simulink library "Enrg_conv_El_to_Mec_Bosch"  (R2016a)
settings: Solver=ode1  StartTime=0.0  StopTime=Inf  FixedStep=0.001  RelTol=1e-3
undefined symbols (not defined in the file): drvEmot_RefTqeMOT, FirstDrivenAxle_FirstDrivenAxleNoOfEmot, FMIKit, SecondDrivenAxle_SecondDrivenAxleNoOfEmot
libraries: Enrg_conv_El_to_Mec_Bosch x13, Electrical_converter x8
(part 2 of 5)

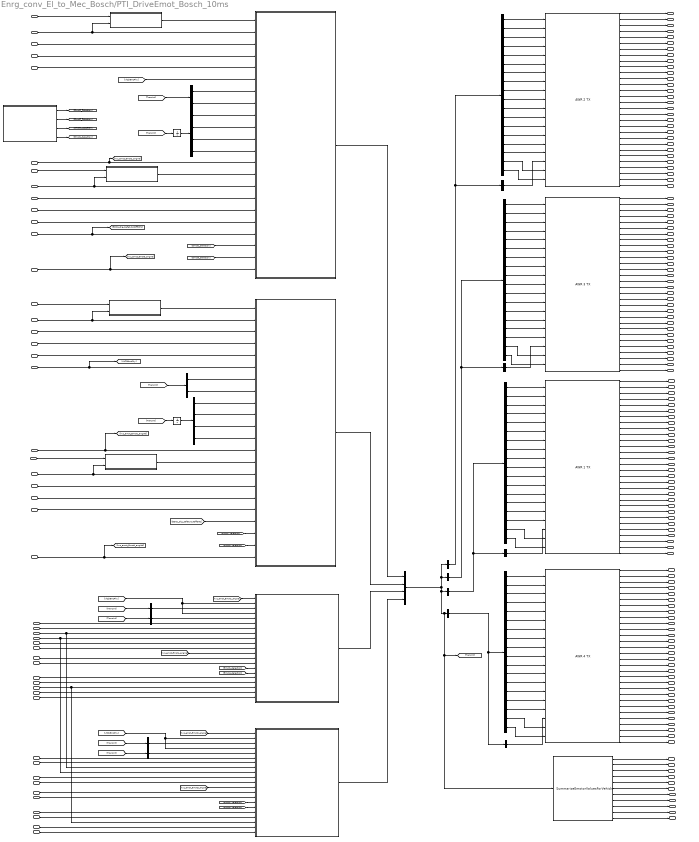
== system Enrg_conv_El_to_Mec_Bosch/PTI_DriveEmot_Bosch_10ms ==
  vltZkBmsPhy : Inport
  HVFreigabeHW1_SiRelay_D : Inport  Port=2
  HVFreigabeHW4_SiRelay_D : Inport  Port=3
  edcu_EMD1_CMD_ClearErrors : Inport  Port=4
  edcu_EMD1_CMD_ControlMode : Inport  Port=5
  edcu_EMD1_CMD_SpeedRefLim : Inport  Port=6
  pti_tqDesired_PTI1 : Inport  Description=[Nm]  Port=7
      settings: AttributesFormatString=%<Description>
  edcu_EMD4_CMD_ClearErrors : Inport  Port=8
  edcu_EMD4_CMD_ControlMode : Inport  Port=9
  edcu_EMD4_CMD_SpeedRefLim : Inport  Port=10
  pti_tqDesired_PTI4 : Inport  Description=[Nm]  Port=11
      settings: AttributesFormatString=%<Description>
  HVFreigabeHW2_SiRelay_D : Inport  Port=12
  HVFreigabeHW3_SiRelay_D : Inport  Port=13
  edcu_EMD2_CMD_ClearErrors : Inport  Port=14
  edcu_EMD2_CMD_ControlMode : Inport  Port=15
  edcu_EMD2_CMD_SpeedRefLim : Inport  Port=16
  pti_tqDesired_PTI2 : Inport  Description=[Nm]  Port=17
      settings: AttributesFormatString=%<Description>
  edcu_EMD3_CMD_ClearErrors : Inport  Port=18
  edcu_EMD3_CMD_ControlMode : Inport  Port=19
  edcu_EMD3_CMD_SpeedRefLim : Inport  Port=20
  pti_tqDesired_PTI3 : Inport  Description=[Nm]  Port=21
      settings: AttributesFormatString=%<Description>
  EDCU_Dig_SafetyCutOffDG1 : Inport  Port=22
  hvs_driveInverter1_switching_frequency : Inport  Port=23
  hvs_driveInverter2_switching_frequency : Inport  Port=24
  hvs_driveInverter3_switching_frequency : Inport  Port=25
  hvs_driveInverter4_switching_frequency : Inport  Port=26
  hvs_emot_Emot1_angVel : Inport  Port=27
  hvs_emot_Emot2_angVel : Inport  Port=28
  hvs_emot_Emot3_angVel : Inport  Port=29
  hvs_emot_Emot4_angVel : Inport  Port=30
  hvs_driveInverter_coolant_temperature : Inport  Port=31
  hvs_drvEmot1_Oil_Temperature : Inport  Port=32
  hvs_drvEmot1_Coolant_Temperature : Inport  Port=33
  hvs_drvEmot4Oil_Temperature : Inport  Port=34
  hvs_drvEmot4_Coolant_Temperature : Inport  Port=35
  hvs_drvEmot2_Oil_Temperature : Inport  Port=36
  hvs_drvEmot2_Coolant_Temperature : Inport  Port=37
  hvs_drvEmot3Oil_Temperature : Inport  Port=38
  hvs_drvEmot3_Coolant_Temperature : Inport  Port=39
  hvs_drvEmot_Ambient_Temperature : Inport  Port=40
  hvs_drvEmot1CoolantFlow_vdot : Inport  Port=41
  hvs_drvEmot1OilFlow_vdot : Inport  Port=42
  hvs_driveInverterCoolantFlow_vdot : Inport  Port=43
  hvs_drvEmot4CoolantFlow_vdot : Inport  Port=44
  hvs_drvEmot4OilFlow_vdot : Inport  Port=45
  hvs_drvEmot2CoolantFlow_vdot : Inport  Port=46
  hvs_drvEmot2OilFlow_vdot : Inport  Port=47
  hvs_drvEmot3CoolantFlow_vdot : Inport  Port=48
  hvs_drvEmot3OilFlow_vdot : Inport  Port=49
  AWR 1 TX1 : Enrg_conv_El_to_Mec_Bosch/PTI_DriveEmot_Bosch/AWR 1 TX
  AWR 2 TX1 : Enrg_conv_El_to_Mec_Bosch/PTI_DriveEmot_Bosch/AWR 2 TX
  AWR 3 TX1 : Enrg_conv_El_to_Mec_Bosch/PTI_DriveEmot_Bosch/AWR 3 TX
  AWR 4 TX1 : Enrg_conv_El_to_Mec_Bosch/PTI_DriveEmot_Bosch/AWR 4 TX
  AWR1_4 : Subsystem
  AWR2_3 : Subsystem
  Bus Selector21 : BusSelector  OutputSignals=EMD2_ACT_DcLinkVoltage,EMD_ACT_DigitalInput1,EMD_ACT_MaximumAvailableTorque,EMD_ACT_DcLinkPower,EMD_ACT_MotorSpeed,EMD_ACT_MotorTorque,EMD_ACT_InverterState,EMD_ACT_ReferenceTorqueLimited,drvEmot_T_Stator,drvEmot_T_Rotor,Inv_Ploss,mot_Ploss,uStator,iStator,modIdx,cosPhi,wasteHeat_coolant,wasteHeat_oil
  Bus Selector22 : BusSelector  OutputSignals=EMD1_ACT_DcLinkVoltage,EMD_ACT_DigitalInput1,EMD_ACT_MaximumAvailableTorque,EMD_ACT_DcLinkPower,EMD_ACT_MotorSpeed,EMD_ACT_MotorTorque,EMD_ACT_InverterState,EMD_ACT_ReferenceTorqueLimited,drvEmot_T_Stator,drvEmot_T_Rotor,Inv_Ploss,mot_Ploss,uStator,iStator,modIdx,cosPhi,wasteHeat_coolant,wasteHeat_oil
  Bus Selector23 : BusSelector  OutputSignals=EMD4_ACT_DcLinkVoltage,EMD_ACT_DigitalInput1,EMD_ACT_MaximumAvailableTorque,EMD_ACT_DcLinkPower,EMD_ACT_MotorSpeed,EMD_ACT_MotorTorque,EMD_ACT_InverterState,EMD_ACT_ReferenceTorqueLimited,drvEmot_T_Stator,drvEmot_T_Rotor,Inv_Ploss,mot_Ploss,uStator,iStator,modIdx,cosPhi,wasteHeat_coolant,wasteHeat_oil
  Bus Selector{24..27} (4 alike) : BusSelector  OutputSignals=driveInverter_Temperatures  OutputAsBus=on
  Bus Selector28 : BusSelector  OutputSignals=EMD3_ACT_DcLinkVoltage,EMD_ACT_DigitalInput1,EMD_ACT_MaximumAvailableTorque,EMD_ACT_DcLinkPower,EMD_ACT_MotorSpeed,EMD_ACT_MotorTorque,EMD_ACT_InverterState,EMD_ACT_ReferenceTorqueLimited,drvEmot_T_Stator,drvEmot_T_Rotor,Inv_Ploss,mot_Ploss,uStator,iStator,modIdx,cosPhi,wasteHeat_oil,wasteHeat_coolant
  Bus Creator : BusCreator  Inputs=4
  Bus Selector1 : BusSelector  OutputSignals=awr1_4B.awr1B.trqEmotDesPhy
  Bus Selector19 : BusSelector  OutputSignals=emot2_3B.emot2B.trqEmotPhy,emot2_3B.emot3B.trqEmotPhy
  Bus Selector2 : BusSelector  OutputSignals=awr1_4B.awr4B.trqEmotDesPhy
  Bus Selector20 : BusSelector  OutputSignals=emot1_4B.emot1B.trqEmotPhy,emot1_4B.emot4B.trqEmotPhy
  Bus Selector29 : BusSelector  OutputSignals=awr2_3B.awr3B.EMD3_ACT_DcLinkVoltage,awr2_3B.awr3B.EMD_ACT_DigitalInput1,awr2_3B.awr3B.EMD_ACT_MaximumAvailableTorque,awr2_3B.awr3B.EMD_ACT_DcLinkPower,awr2_3B.awr3B.EMD_ACT_MotorSpeed,awr2_3B.awr3B.EMD_ACT_MotorTorque,awr2_3B.awr3B.EMD_ACT_InverterState,awr2_3B.awr3B.EMD_ACT_ReferenceTorqueLimited,awr2_3B.awr3B.trqEmotDesPhy,emot2_3B.emot3B.driveInverter_Temperatures,emot2_3B.emot3B.drvEmot_T_Stator,emot2_3B.emot3B.drvEmot_T_Rotor,emot2_3B.emot3B.Inv_Ploss,emot2_3B.emot3B.mot_Ploss,emot2_3B.emot3B.uStator,emot2_3B.emot3B.iStator,emot2_3B.emot3B.modIdx,emot2_3B.emot3B.cosPhi,emot2_3B.emot3B.wasteHeat_coolant,emot2_3B.emot3B.wasteHeat_oil  OutputAsBus=on
  Bus Selector3 : BusSelector  OutputSignals=emot2_3B.emot2B.pwrEmotPhy,emot2_3B.emot3B.pwrEmotPhy,emot2_3B.emot2B.trqEmotMax,emot2_3B.emot3B.trqEmotMax
  Bus Selector30 : BusSelector  OutputSignals=awr2_3B.awr2B.EMD2_ACT_DcLinkVoltage,awr2_3B.awr2B.EMD_ACT_DigitalInput1,awr2_3B.awr2B.EMD_ACT_MaximumAvailableTorque,awr2_3B.awr2B.EMD_ACT_DcLinkPower,awr2_3B.awr2B.EMD_ACT_MotorSpeed,awr2_3B.awr2B.EMD_ACT_MotorTorque,awr2_3B.awr2B.EMD_ACT_InverterState,awr2_3B.awr2B.EMD_ACT_ReferenceTorqueLimited,awr2_3B.awr2B.trqEmotDesPhy,emot2_3B.emot2B.driveInverter_Temperatures,emot2_3B.emot2B.drvEmot_T_Stator,emot2_3B.emot2B.drvEmot_T_Rotor,emot2_3B.emot2B.Inv_Ploss,emot2_3B.emot2B.mot_Ploss,emot2_3B.emot2B.uStator,emot2_3B.emot2B.iStator,emot2_3B.emot2B.modIdx,emot2_3B.emot2B.cosPhi,emot2_3B.emot2B.wasteHeat_coolant,emot2_3B.emot2B.wasteHeat_oil  OutputAsBus=on
  Bus Selector31 : BusSelector  OutputSignals=awr1_4B.awr4B.EMD4_ACT_DcLinkVoltage,awr1_4B.awr4B.EMD_ACT_DigitalInput1,awr1_4B.awr4B.EMD_ACT_MaximumAvailableTorque,awr1_4B.awr4B.EMD_ACT_DcLinkPower,awr1_4B.awr4B.EMD_ACT_MotorSpeed,awr1_4B.awr4B.EMD_ACT_MotorTorque,awr1_4B.awr4B.EMD_ACT_InverterState,awr1_4B.awr4B.EMD_ACT_ReferenceTorqueLimited,awr1_4B.awr4B.trqEmotDesPhy,emot1_4B.emot4B.driveInverter_Temperatures,emot1_4B.emot4B.drvEmot_T_Stator,emot1_4B.emot4B.drvEmot_T_Rotor,emot1_4B.emot4B.Inv_Ploss,emot1_4B.emot4B.mot_Ploss,emot1_4B.emot4B.uStator,emot1_4B.emot4B.iStator,emot1_4B.emot4B.modIdx,emot1_4B.emot4B.cosPhi,emot1_4B.emot4B.wasteHeat_coolant,emot1_4B.emot4B.wasteHeat_oil  OutputAsBus=on
  Bus Selector32 : BusSelector  OutputSignals=awr1_4B.awr1B.EMD1_ACT_DcLinkVoltage,awr1_4B.awr1B.EMD_ACT_DigitalInput1,awr1_4B.awr1B.EMD_ACT_MaximumAvailableTorque,awr1_4B.awr1B.EMD_ACT_DcLinkPower,awr1_4B.awr1B.EMD_ACT_MotorSpeed,awr1_4B.awr1B.EMD_ACT_MotorTorque,awr1_4B.awr1B.EMD_ACT_InverterState,awr1_4B.awr1B.EMD_ACT_ReferenceTorqueLimited,awr1_4B.awr1B.trqEmotDesPhy,emot1_4B.emot1B.driveInverter_Temperatures,emot1_4B.emot1B.drvEmot_T_Stator,emot1_4B.emot1B.drvEmot_T_Rotor,emot1_4B.emot1B.Inv_Ploss,emot1_4B.emot1B.mot_Ploss,emot1_4B.emot1B.uStator,emot1_4B.emot1B.iStator,emot1_4B.emot1B.modIdx,emot1_4B.emot1B.cosPhi,emot1_4B.emot1B.wasteHeat_coolant,emot1_4B.emot1B.wasteHeat_oil  OutputAsBus=on
  Bus Selector4 : BusSelector  OutputSignals=emot1_4B.emot1B.pwrEmotPhy,emot1_4B.emot4B.pwrEmotPhy,emot1_4B.emot1B.trqEmotMax,emot1_4B.emot4B.trqEmotMax
  Bus Selector7 : BusSelector  OutputSignals=awr2_3B.awr2B.trqEmotDesPhy
  Bus Selector8 : BusSelector  OutputSignals=awr2_3B.awr3B.trqEmotDesPhy
  EMD1_CMD_Command : Subsystem
  EMD1_CMD_Command1 : Subsystem
  EMD1_CMD_Command2 : Subsystem
  EMD1_CMD_Command3 : Subsystem
  Emot1_4 : Subsystem
  Emot2_3 : Subsystem
  MotorSelection : Subsystem
  SummarizeEmotorValuesForVehicle1 : Enrg_conv_El_to_Mec_Bosch/PTI_DriveEmot_Bosch/SummarizeEmotorValuesForVehicle
  Unit Delay2 : UnitDelay  SampleTime=-1
  Unit Delay3 : UnitDelay  SampleTime=-1
  hvs_dcLink_drive_emot_current1 : Outport
  hvs_emot_Emot1_torque1 : Outport  Port=2
  hvs_emot_Emot2_torque1 : Outport  Port=3
  hvs_emot_Emot3_torque1 : Outport  Port=4
  hvs_emot_Emot4_torque1 : Outport  Port=5
  hvs_driveInverter_wasteHeat_power1 : Outport  Port=6
  hvs_drvEmotWasteHeat_power1 : Outport  Port=7
  hvs_drvEmot1WasteHeat_power1 : Outport  Port=8
  hvs_drvEmot2WasteHeat_power1 : Outport  Port=9
  hvs_drvEmot3WasteHeat_power1 : Outport  Port=10
  hvs_drvEmot4WasteHeat_power1 : Outport  Port=11
  hvs_EMD1_ACT_DigitalInput2 : Outport  Port=12
  hvs_EMD1_ACT_InverterState1 : Outport  Port=13
  hvs_EMD1_ACT_MaxAvailableTorque1 : Outport  Port=14
  hvs_EMD1_ACT_ReferenceTorqueLim1 : Outport  Port=15
  hvs_EMD1_ACT_Torque1 : Outport  Port=16
  hvs_EMD1_ACT_DcLinkPower1 : Outport  Port=17
  hvs_EMD1_ACT_MotorSpeed1 : Outport  Port=18
  hvs_EMD1_ACT_DcLinkVoltage1 : Outport  Port=19
  hvs_EMD1_ACT_MaxJunctionTemp1 : Outport  Port=20
  hvs_EMD1_ACT_MotorTemperature1 : Outport  Port=21
  hvs_EMD1_ACT_RotorTemperature1 : Outport  Port=22
  hvs_EMD1_ACT_InverterLosses1 : Outport  Port=23
  hvs_EMD1_ACT_MotorLosses1 : Outport  Port=24
  hvs_EMD1_uStator1 : Outport  Port=25
  hvs_EMD1_iStator1 : Outport  Port=26
  hvs_EMD1_modIdx1 : Outport  Port=27
  hvs_EMD1_cosPhi1 : Outport  Port=28
  hvs_EMD1_ACT_tSnsrPwrModlMax1 : Outport  Port=29
  hvs_EMD1_ACT_tCapSnsr1 : Outport  Port=30
  hvs_EMD1_ACT_tCapCoil1 : Outport  Port=31
  hvs_EMD1_ACT_tCapAcCnctr1 : Outport  Port=32
  hvs_EMD1_ACT_tCapDcCnctr1 : Outport  Port=33
  hvs_EMD1_ACT_tIvtrAcRail1 : Outport  Port=34
  hvs_EMD1_ACT_tIvtrDcRail1 : Outport  Port=35
  hvs_EMD1_ACT_tIvtrAcRailIphaSnsr1 : Outport  Port=36
  hvs_EMD1_ACT_tIvtrDcRailCnctr1 : Outport  Port=37
  hvs_EMD1_ACT_tCoolIvtrOuttk1 : Outport  Port=38
  hvs_EMD4_ACT_DigitalInput2 : Outport  Port=39
  hvs_EMD4_ACT_InverterState1 : Outport  Port=40
  hvs_EMD4_ACT_MaxAvailableTorque1 : Outport  Port=41
  hvs_EMD4_ACT_ReferenceTorqueLim1 : Outport  Port=42
  hvs_EMD4_ACT_Torque1 : Outport  Port=43
  hvs_EMD4_ACT_DcLinkPower1 : Outport  Port=44
  hvs_EMD4_ACT_MotorSpeed1 : Outport  Port=45
  hvs_EMD4_ACT_DcLinkVoltage1 : Outport  Port=46
  hvs_EMD4_ACT_MaxJunctionTemperature1 : Outport  Port=47
  hvs_EMD4_ACT_MotorTemperature1 : Outport  Port=48
  hvs_EMD4_ACT_RotorTemperature1 : Outport  Port=49
  hvs_EMD4_ACT_InverterLosses1 : Outport  Port=50
  hvs_EMD4_ACT_MotorLosses1 : Outport  Port=51
  hvs_EMD4_uStator1 : Outport  Port=52
  hvs_EMD4_iStator1 : Outport  Port=53
  hvs_EMD4_modIdx1 : Outport  Port=54
  hvs_EMD4_cosPhi1 : Outport  Port=55
  hvs_EMD4_ACT_tSnsrPwrModlMax1 : Outport  Port=56
  hvs_EMD4_ACT_tCapSnsr1 : Outport  Port=57
  hvs_EMD4_ACT_tCapCoil1 : Outport  Port=58
  hvs_EMD4_ACT_tCapAcCnctr1 : Outport  Port=59
  hvs_EMD4_ACT_tCapDcCnctr1 : Outport  Port=60
  hvs_EMD4_ACT_tIvtrAcRail1 : Outport  Port=61
  hvs_EMD4_ACT_tIvtrDcRail1 : Outport  Port=62
  hvs_EMD4_ACT_tIvtrAcRailIphaSnsr1 : Outport  Port=63
  hvs_EMD4_ACT_tIvtrDcRailCnctr1 : Outport  Port=64
  hvs_EMD4_ACT_tCoolIvtrOuttk1 : Outport  Port=65
  hvs_EMD3_ACT_DigitalInput2 : Outport  Port=66
  hvs_EMD3_ACT_InverterState1 : Outport  Port=67
  hvs_EMD3_ACT_MaxAvailableTorque1 : Outport  Port=68
  hvs_EMD3_ACT_ReferenceTorqueLim1 : Outport  Port=69
  hvs_EMD3_ACT_Torque1 : Outport  Port=70
  hvs_EMD3_ACT_DcLinkPower1 : Outport  Port=71
  hvs_EMD3_ACT_MotorSpeed1 : Outport  Port=72
  hvs_EMD3_ACT_DcLinkVoltage1 : Outport  Port=73
  hvs_EMD3_ACT_MaxJunctionTemp1 : Outport  Port=74
  hvs_EMD3_ACT_MotorTemperature1 : Outport  Port=75
  hvs_EMD3_ACT_RotorTemperature1 : Outport  Port=76
  hvs_EMD3_ACT_InverterLosses1 : Outport  Port=77
  hvs_EMD3_ACT_MotorLosses1 : Outport  Port=78
  hvs_EMD3_uStator1 : Outport  Port=79
  hvs_EMD3_iStator1 : Outport  Port=80
  hvs_EMD3_modIdx1 : Outport  Port=81
  hvs_EMD3_cosPhi1 : Outport  Port=82
  hvs_EMD3_ACT_tSnsrPwrModlMax1 : Outport  Port=83
  hvs_EMD3_ACT_tCapSnsr1 : Outport  Port=84
  hvs_EMD3_ACT_tCapCoil1 : Outport  Port=85
  hvs_EMD3_ACT_tCapAcCnctr1 : Outport  Port=86
  hvs_EMD3_ACT_tCapDcCnctr1 : Outport  Port=87
  hvs_EMD3_ACT_tIvtrAcRail1 : Outport  Port=88
  hvs_EMD3_ACT_tIvtrDcRail1 : Outport  Port=89
  hvs_EMD3_ACT_tIvtrAcRailIphaSnsr1 : Outport  Port=90
  hvs_EMD3_ACT_tIvtrDcRailCnctr1 : Outport  Port=91
  hvs_EMD3_ACT_tCoolIvtrOuttk1 : Outport  Port=92
  hvs_EMD2_ACT_DigitalInput2 : Outport  Port=93
  hvs_EMD2_ACT_InverterState1 : Outport  Port=94
  hvs_EMD2_ACT_MaxAvailableTorque1 : Outport  Port=95
  hvs_EMD2_ACT_ReferenceTorqueLim1 : Outport  Port=96
  hvs_EMD2_ACT_Torque1 : Outport  Port=97
  hvs_EMD2_ACT_DcLinkPower1 : Outport  Port=98
  hvs_EMD2_ACT_MotorSpeed1 : Outport  Port=99
  hvs_EMD2_ACT_DcLinkVoltage1 : Outport  Port=100
  hvs_EMD2_ACT_MaxJunctionTemp1 : Outport  Port=101
  hvs_EMD2_ACT_MotorTemperature1 : Outport  Port=102
  hvs_EMD2_ACT_RotorTemperature1 : Outport  Port=103
  hvs_EMD2_ACT_InverterLosses1 : Outport  Port=104
  hvs_EMD2_ACT_MotorLosses1 : Outport  Port=105
  hvs_EMD2_uStator1 : Outport  Port=106
  hvs_EMD2_iStator1 : Outport  Port=107
  hvs_EMD2_modIdx1 : Outport  Port=108
  hvs_EMD2_cosPhi1 : Outport  Port=109
  hvs_EMD2_ACT_tSnsrPwrModlMax1 : Outport  Port=110
  hvs_EMD2_ACT_tCapSnsr1 : Outport  Port=111
  hvs_EMD2_ACT_tCapCoil1 : Outport  Port=112
  hvs_EMD2_ACT_tCapAcCnctr1 : Outport  Port=113
  hvs_EMD2_ACT_tCapDcCnctr1 : Outport  Port=114
  hvs_EMD2_ACT_tIvtrAcRail1 : Outport  Port=115
  hvs_EMD2_ACT_tIvtrDcRail1 : Outport  Port=116
  hvs_EMD2_ACT_tIvtrAcRailIphaSnsr1 : Outport  Port=117
  hvs_EMD2_ACT_tIvtrDcRailCnctr1 : Outport  Port=118
  hvs_EMD2_ACT_tCoolIvtrOuttk1 : Outport  Port=119
  hvs_EMD2_ACT_Torque_Nm1 : Outport  Port=120
  hvs_EMD3_ACT_Torque_Nm1 : Outport  Port=121
  hvs_EMD1_ACT_Torque_Nm1 : Outport  Port=122
  hvs_EMD4_ACT_Torque_Nm1 : Outport  Port=123
  hvs_drvEmot2WasteHeatcoolant_power : Outport  Port=124
  hvs_drvEmot2WasteHeatoil_power : Outport  Port=125
  hvs_drvEmot3WasteHeatcoolant_power : Outport  Port=126
  hvs_drvEmot3WasteHeatoil_power : Outport  Port=127
  hvs_drvEmot1WasteHeatcoolant_power : Outport  Port=128
  hvs_drvEmot1WasteHeatoil_power : Outport  Port=129
  hvs_drvEmot4WasteHeatcoolant_power : Outport  Port=130
  hvs_drvEmot4WasteHeatoil_power : Outport  Port=131
  wires:
  hvs_driveInverter2_switching_frequency/1 -> Emot2_3/10(inv2_switching_freq)
  hvs_driveInverter3_switching_frequency/1 -> Emot2_3/11(inv3_switching_freq)
  hvs_driveInverter4_switching_frequency/1 -> Emot1_4/11(inv4_switching_freq)
  hvs_drvEmot3_Coolant_Temperature/1 -> Emot2_3/14(drvEmot3_Coolant_Temperature)
  hvs_drvEmot4_Coolant_Temperature/1 -> Emot1_4/14(drvEmot4_Coolant_Temperature)
  hvs_drvEmot2_Coolant_Temperature/1 -> Emot2_3/7(drvEmot2_Coolant_Temperature)
  hvs_driveInverter1_switching_frequency/1 -> Emot1_4/10(inv1_switching_freq)
  hvs_drvEmot_Ambient_Temperature/1 -> Emot1_4/8(drvEmot_Ambient_Temperature), Emot2_3/8(drvEmot_Ambient_Temperature)
  hvs_drvEmot1_Coolant_Temperature/1 -> Emot1_4/7(drvEmot1_Coolant_Temperature)
  hvs_drvEmot3Oil_Temperature/1 -> Emot2_3/13(drvEmot3_Oil_Temperature)
  hvs_drvEmot2_Oil_Temperature/1 -> Emot2_3/6(drvEmot2_Oil_Temperature)
  hvs_drvEmot4Oil_Temperature/1 -> Emot1_4/13(drvEmot4_Oil_Temperature)
  [hvs_emot_Emot3_angVel] -> Emot2_3/12(emot_Emot3_angVel)
  [hvs_emot_Emot4_angVel] -> Emot1_4/12(emot_Emot4_angVel)
  hvs_emot_Emot4_angVel/1 -> AWR1_4/22(hvs_emot_Emot4_angVel), [hvs_emot_Emot4_angVel]
  hvs_emot_Emot3_angVel/1 -> AWR2_3/22(hvs_emot_Emot3_angVel), [hvs_emot_Emot3_angVel]
  [Emot3_Selection] -> Emot2_3/16(Emot3_Selection)
  [Emot2_Selection] -> Emot2_3/15(Emot2_Selection)
  [Emot4_Selection] -> Emot1_4/16(Emot4_Selection)
  [Emot1_Selection] -> Emot1_4/15(Emot1_Selection)
  [Emot4_Selection] -> AWR1_4/21(Emot4_Selection)
  [Emot1_Selection] -> AWR1_4/20(Emot1_Selection)
  [Emot3_Selection] -> AWR2_3/21(Emot3_Selection)
  [Emot2_Selection] -> AWR2_3/20(Emot2_Selection)
  MotorSelection/4(Emot4_Selection) -> [Emot4_Selection]
  MotorSelection/3(Emot3_Selection) -> [Emot3_Selection]
  MotorSelection/2(Emot2_Selection) -> [Emot2_Selection]
  MotorSelection/1(Emot1_Selection) -> [Emot1_Selection]
  Bus Selector3/4 -> AWR2_3/12(trqEmot3Max)  "<trqEmotMax>"
  Bus Selector3/3 -> AWR2_3/11(trqEmot2Max)  "<trqEmotMax>"
  Bus Selector3/2 -> AWR2_3/10(pwEmot3Phy)  "<pwrEmotPhy>"
  Bus Selector3/1 -> AWR2_3/9(pwEmot2Phy)  "<pwrEmotPhy>"
  Bus Selector4/4 -> AWR1_4/12(trqEmot4Max)  "<trqEmotMax>"
  Bus Selector4/3 -> AWR1_4/11(trqEmot1Max)  "<trqEmotMax>"
  Bus Selector4/2 -> AWR1_4/10(pwEmot4Phy)  "<pwrEmotPhy>"
  Bus Selector4/1 -> AWR1_4/9(pwEmot1Phy)  "<pwrEmotPhy>"
  [EDCU_Dig_SafetyCutOffDG1] -> AWR1_4/19(EDCU_Dig_SafetyCutOffDG1)
  EDCU_Dig_SafetyCutOffDG1/1 -> AWR2_3/19(EDCU_Dig_SafetyCutOffDG1), [EDCU_Dig_SafetyCutOffDG1]
  Emot2_3/1(emot2_3B) -> Bus Creator/4
  Bus Selector8/1 -> Emot2_3/5(trqEmotDesPhy3)  "<trqEmotDesPhy>"
  [vltZkBmsPhy] -> Emot2_3/4(voltBatHV3), Emot2_3/2(voltBatHV2)
  Bus Selector7/1 -> Emot2_3/3(trqEmotDesPhy2)  "<trqEmotDesPhy>"
  [hvs_emot_Emot2_angVel] -> Emot2_3/1(emot_Emot2_angVel)
  [TransInt] -> Bus Selector8/1
  [TransInt] -> Bus Selector7/1
  AWR2_3/1(awr2_3B) -> Bus Creator/1
  Emot1_4/1(emot1_4B) -> Bus Creator/3
  Bus Selector2/1 -> Emot1_4/5(trqEmotDesPhy4)  "<trqEmotDesPhy>"
  [vltZkBmsPhy] -> Emot1_4/4(voltBatHV4), Emot1_4/2(voltBatHV1)
  Bus Selector1/1 -> Emot1_4/3(trqEmotDesPhy1)  "<trqEmotDesPhy>"
  [hvs_emot_Emot1_angVel] -> Emot1_4/1(emot_Emot1_angVel)
  hvs_emot_Emot2_angVel/1 -> AWR2_3/13(hvs_emot_Emot2_angVel), [hvs_emot_Emot2_angVel]
  [vltZkBmsPhy] -> AWR2_3/6(vltZkBmsPhy)
  HVFreigabeHW3_SiRelay_D/1 -> AWR2_3/18(HVFreigabeHW3_SiRelay_D)
  pti_tqDesired_PTI3/1 -> AWR2_3/17(EMD3_CMD_TorqueRefLim)
  edcu_EMD3_CMD_SpeedRefLim/1 -> AWR2_3/16(EMD3_CMD_SpeedRefLim)
  EMD1_CMD_Command3/1(Out_EMD1_CMD_Command) -> AWR2_3/14(EMD3_CMD_Commamd)
  HVFreigabeHW2_SiRelay_D/1 -> AWR2_3/5(HVFreigabeHW2_SiRelay_D)
  pti_tqDesired_PTI2/1 -> AWR2_3/4(EMD2_CMD_TorqueRefLim)
  edcu_EMD2_CMD_SpeedRefLim/1 -> AWR2_3/3(EMD2_CMD_SpeedRefLim)
  EMD1_CMD_Command2/1(Out_EMD1_CMD_Command) -> AWR2_3/1(EMD2_CMD_Commamd)
  Unit Delay2/1 -> Bus Selector3/1
  [TransInt] -> Unit Delay2/1
  edcu_EMD3_CMD_ClearErrors/1 -> EMD1_CMD_Command3/1(EMD1_CMD_ClearErrors)
  edcu_EMD3_CMD_ControlMode/1 -> AWR2_3/15(EMD3_CMD_MotorControlMode), EMD1_CMD_Command3/2(EMD1_CMD_MotorControlMode)
  edcu_EMD2_CMD_ClearErrors/1 -> EMD1_CMD_Command2/1(EMD1_CMD_ClearErrors)
  edcu_EMD2_CMD_ControlMode/1 -> AWR2_3/2(EMD2_CMD_MotorControlMode), EMD1_CMD_Command2/2(EMD1_CMD_MotorControlMode)
  AWR1_4/1(awr1_4B) -> Bus Creator/2
  HVFreigabeHW4_SiRelay_D/1 -> AWR1_4/18(HVFreigabeHW4_SiRelay_D)
  pti_tqDesired_PTI4/1 -> AWR1_4/17(EMD4_CMD_TorqueRefLim)
  edcu_EMD4_CMD_SpeedRefLim/1 -> AWR1_4/16(EMD4_CMD_SpeedRefLim)
  EMD1_CMD_Command1/1(Out_EMD1_CMD_Command) -> AWR1_4/14(EMD4_CMD_Commamd)
  HVFreigabeHW1_SiRelay_D/1 -> AWR1_4/5(HVFreigabeHW_SiRelay_D)
  pti_tqDesired_PTI1/1 -> AWR1_4/4(EMD1_CMD_TorqueRefLim)
  edcu_EMD1_CMD_SpeedRefLim/1 -> AWR1_4/3(EMD1_CMD_SpeedRefLim)
  EMD1_CMD_Command/1(Out_EMD1_CMD_Command) -> AWR1_4/1(EMD1_CMD_Commamd)
  Unit Delay3/1 -> Bus Selector4/1
  [TransInt] -> Unit Delay3/1
  [TransInt] -> Bus Selector2/1
  [TransInt] -> Bus Selector1/1
  edcu_EMD4_CMD_ClearErrors/1 -> EMD1_CMD_Command1/1(EMD1_CMD_ClearErrors)
  edcu_EMD4_CMD_ControlMode/1 -> AWR1_4/15(EMD4_CMD_MotorControlMode), EMD1_CMD_Command1/2(EMD1_CMD_MotorControlMode)
  hvs_emot_Emot1_angVel/1 -> AWR1_4/13(hvs_emot_Emot1_angVel), [hvs_emot_Emot1_angVel]
  vltZkBmsPhy/1 -> AWR1_4/6(vltZkBmsPhy), [vltZkBmsPhy]
  edcu_EMD1_CMD_ClearErrors/1 -> EMD1_CMD_Command/1(EMD1_CMD_ClearErrors)
  edcu_EMD1_CMD_ControlMode/1 -> AWR1_4/2(EMD1_CMD_MotorControlMode), EMD1_CMD_Command/2(EMD1_CMD_MotorControlMode)
  hvs_drvEmot1_Oil_Temperature/1 -> Emot1_4/6(drvEmot1_Oil_Temperature)
  hvs_driveInverter_coolant_temperature/1 -> Emot1_4/9(inv_coolant_temperature), Emot2_3/9(inv_coolant_temperature)
  [TransInt] -> Bus Selector19/1
  Bus Selector19/1 -> AWR2_3/7(trqEmot2Phy)  "<trqEmotPhy>"
  Bus Selector19/2 -> AWR2_3/8(trqEmot3Phy)  "<trqEmotPhy>"
  [TransInt] -> Bus Selector20/1
  Bus Selector20/1 -> AWR1_4/7(trqEmot1Phy)  "<trqEmotPhy>"
  Bus Selector20/2 -> AWR1_4/8(trqEmot4Phy)  "<trqEmotPhy>"
  hvs_drvEmot1CoolantFlow_vdot/1 -> Emot1_4/17(drvEmot1CoolantFlow_vdot)
  hvs_drvEmot1OilFlow_vdot/1 -> Emot1_4/18(drvEmot1OilFlow_vdot)
  hvs_driveInverterCoolantFlow_vdot/1 -> Emot2_3/19(driveInverterCoolantFlow_vdot), Emot1_4/19(driveInverterCoolantFlow_vdot)
  hvs_drvEmot4CoolantFlow_vdot/1 -> Emot1_4/20(drvEmot4CoolantFlow_vdot)
  hvs_drvEmot4OilFlow_vdot/1 -> Emot1_4/21(drvEmot4OilFlow_vdot)
  hvs_drvEmot2OilFlow_vdot/1 -> Emot2_3/18(drvEmot2OilFlow_vdot)
  hvs_drvEmot2CoolantFlow_vdot/1 -> Emot2_3/17(drvEmot2CoolantFlow_vdot)
  hvs_drvEmot3CoolantFlow_vdot/1 -> Emot2_3/20(drvEmot3CoolantFlow_vdot)
  hvs_drvEmot3OilFlow_vdot/1 -> Emot2_3/21(drvEmot3OilFlow_vdot)
  Bus Selector31/1 -> Bus Selector23/1, Bus Selector27/1  "TransInt"
  Bus Creator/1 -> [TransInt], SummarizeEmotorValuesForVehicle1/1, Bus Selector31/1, Bus Selector32/1, Bus Selector30/1, Bus Selector29/1  "TransInt"
  Bus Selector32/1 -> Bus Selector22/1, Bus Selector26/1  "TransInt"
  SummarizeEmotorValuesForVehicle1/1 -> hvs_emot_Emot1_torque1/1
  SummarizeEmotorValuesForVehicle1/7 -> hvs_dcLink_drive_emot_current1/1
  SummarizeEmotorValuesForVehicle1/6 -> hvs_drvEmotWasteHeat_power1/1
  SummarizeEmotorValuesForVehicle1/5 -> hvs_driveInverter_wasteHeat_power1/1
  Bus Selector29/1 -> Bus Selector28/1, Bus Selector25/1  "TransInt"
  Bus Selector30/1 -> Bus Selector21/1, Bus Selector24/1  "TransInt"
  AWR 2 TX1/1 -> hvs_EMD2_ACT_DigitalInput2/1
  AWR 2 TX1/2 -> hvs_EMD2_ACT_InverterState1/1
  AWR 2 TX1/3 -> hvs_EMD2_ACT_MaxAvailableTorque1/1
  AWR 2 TX1/4 -> hvs_EMD2_ACT_ReferenceTorqueLim1/1
  AWR 2 TX1/5 -> hvs_EMD2_ACT_Torque1/1
  AWR 2 TX1/6 -> hvs_EMD2_ACT_DcLinkPower1/1
  AWR 2 TX1/7 -> hvs_EMD2_ACT_MotorSpeed1/1
  AWR 2 TX1/8 -> hvs_EMD2_ACT_DcLinkVoltage1/1
  AWR 2 TX1/17 -> hvs_EMD2_ACT_MaxJunctionTemp1/1
  AWR 2 TX1/9 -> hvs_EMD2_ACT_MotorTemperature1/1
  SummarizeEmotorValuesForVehicle1/2 -> hvs_emot_Emot2_torque1/1
  AWR 2 TX1/11 -> hvs_EMD2_ACT_InverterLosses1/1
  AWR 2 TX1/12 -> hvs_EMD2_ACT_MotorLosses1/1
  SummarizeEmotorValuesForVehicle1/3 -> hvs_emot_Emot3_torque1/1
  SummarizeEmotorValuesForVehicle1/4 -> hvs_emot_Emot4_torque1/1
  SummarizeEmotorValuesForVehicle1/8 -> hvs_drvEmot1WasteHeat_power1/1
  SummarizeEmotorValuesForVehicle1/9 -> hvs_drvEmot2WasteHeat_power1/1
  SummarizeEmotorValuesForVehicle1/10 -> hvs_drvEmot3WasteHeat_power1/1
  SummarizeEmotorValuesForVehicle1/11 -> hvs_drvEmot4WasteHeat_power1/1
  AWR 2 TX1/10 -> hvs_EMD2_ACT_RotorTemperature1/1
  AWR 2 TX1/13 -> hvs_EMD2_uStator1/1
  AWR 2 TX1/14 -> hvs_EMD2_iStator1/1
  Bus Selector28/6 -> AWR 3 TX1/6  "<EMD_ACT_MotorTorque>"
  Bus Selector28/1 -> AWR 3 TX1/1  "<EMD3_ACT_DcLinkVoltage>"
  Bus Selector28/2 -> AWR 3 TX1/2  "<EMD_ACT_DigitalInput1>"
  Bus Selector28/4 -> AWR 3 TX1/4  "<EMD_ACT_DcLinkPower>"
  Bus Selector28/5 -> AWR 3 TX1/5  "<EMD_ACT_MotorSpeed>"
  Bus Selector28/7 -> AWR 3 TX1/7  "<EMD_ACT_InverterState>"
  Bus Selector28/8 -> AWR 3 TX1/8  "<EMD_ACT_ReferenceTorqueLimited>"
  Bus Selector28/3 -> AWR 3 TX1/3  "<EMD_ACT_MaximumAvailableTorque>"
  Bus Selector28/9 -> AWR 3 TX1/9  "<drvEmot_T_Stator>"
  Bus Selector28/10 -> AWR 3 TX1/10  "<drvEmot_T_Rotor>"
  Bus Selector28/12 -> AWR 3 TX1/12  "<mot_Ploss>"
  Bus Selector28/13 -> AWR 3 TX1/13  "<uStator>"
  Bus Selector28/11 -> AWR 3 TX1/11  "<Inv_Ploss>"
  Bus Selector28/14 -> AWR 3 TX1/14  "<iStator>"
  Bus Selector21/5 -> AWR 2 TX1/5  "<EMD_ACT_MotorSpeed>"
  Bus Selector21/6 -> AWR 2 TX1/6  "<EMD_ACT_MotorTorque>"
  Bus Selector21/2 -> AWR 2 TX1/2  "<EMD_ACT_DigitalInput1>"
  Bus Selector21/12 -> AWR 2 TX1/12  "<mot_Ploss>"
  Bus Selector21/8 -> AWR 2 TX1/8  "<EMD_ACT_ReferenceTorqueLimited>"
  Bus Selector21/9 -> AWR 2 TX1/9  "<drvEmot_T_Stator>"
  Bus Selector21/14 -> AWR 2 TX1/14  "<iStator>"
  Bus Selector21/3 -> AWR 2 TX1/3  "<EMD_ACT_MaximumAvailableTorque>"
  Bus Selector21/7 -> AWR 2 TX1/7  "<EMD_ACT_InverterState>"
  Bus Selector21/4 -> AWR 2 TX1/4  "<EMD_ACT_DcLinkPower>"
  Bus Selector21/10 -> AWR 2 TX1/10  "<drvEmot_T_Rotor>"
  Bus Selector21/1 -> AWR 2 TX1/1  "<EMD2_ACT_DcLinkVoltage>"
  Bus Selector21/11 -> AWR 2 TX1/11  "<Inv_Ploss>"
  Bus Selector21/13 -> AWR 2 TX1/13  "<uStator>"
  Bus Selector24/1 -> AWR 2 TX1/17  "driveInverter_Temperatures_Bus"
  AWR 2 TX1/18 -> hvs_EMD2_ACT_tSnsrPwrModlMax1/1
  AWR 2 TX1/19 -> hvs_EMD2_ACT_tCapSnsr1/1
  AWR 2 TX1/20 -> hvs_EMD2_ACT_tCapCoil1/1
  AWR 2 TX1/21 -> hvs_EMD2_ACT_tCapAcCnctr1/1
  AWR 2 TX1/22 -> hvs_EMD2_ACT_tCapDcCnctr1/1
  AWR 2 TX1/23 -> hvs_EMD2_ACT_tIvtrAcRail1/1
  AWR 2 TX1/24 -> hvs_EMD2_ACT_tIvtrDcRail1/1
  AWR 2 TX1/25 -> hvs_EMD2_ACT_tIvtrAcRailIphaSnsr1/1
  AWR 2 TX1/26 -> hvs_EMD2_ACT_tIvtrDcRailCnctr1/1
  AWR 2 TX1/27 -> hvs_EMD2_ACT_tCoolIvtrOuttk1/1
  Bus Selector25/1 -> AWR 3 TX1/17  "driveInverter_Temperatures_Bus"
  AWR 3 TX1/1 -> hvs_EMD3_ACT_DigitalInput2/1
  AWR 3 TX1/2 -> hvs_EMD3_ACT_InverterState1/1
  AWR 3 TX1/3 -> hvs_EMD3_ACT_MaxAvailableTorque1/1
  AWR 3 TX1/4 -> hvs_EMD3_ACT_ReferenceTorqueLim1/1
  AWR 3 TX1/5 -> hvs_EMD3_ACT_Torque1/1
  AWR 3 TX1/6 -> hvs_EMD3_ACT_DcLinkPower1/1
  AWR 3 TX1/7 -> hvs_EMD3_ACT_MotorSpeed1/1
  AWR 3 TX1/8 -> hvs_EMD3_ACT_DcLinkVoltage1/1
  AWR 3 TX1/9 -> hvs_EMD3_ACT_MotorTemperature1/1
  AWR 3 TX1/10 -> hvs_EMD3_ACT_RotorTemperature1/1
  AWR 3 TX1/11 -> hvs_EMD3_ACT_InverterLosses1/1
  AWR 3 TX1/12 -> hvs_EMD3_ACT_MotorLosses1/1
  AWR 3 TX1/13 -> hvs_EMD3_uStator1/1
  AWR 3 TX1/14 -> hvs_EMD3_iStator1/1
  AWR 3 TX1/17 -> hvs_EMD3_ACT_MaxJunctionTemp1/1
  AWR 3 TX1/18 -> hvs_EMD3_ACT_tSnsrPwrModlMax1/1
  AWR 3 TX1/19 -> hvs_EMD3_ACT_tCapSnsr1/1
  AWR 3 TX1/20 -> hvs_EMD3_ACT_tCapCoil1/1
  AWR 3 TX1/21 -> hvs_EMD3_ACT_tCapAcCnctr1/1
  AWR 3 TX1/22 -> hvs_EMD3_ACT_tCapDcCnctr1/1
  AWR 3 TX1/23 -> hvs_EMD3_ACT_tIvtrAcRail1/1
  AWR 3 TX1/24 -> hvs_EMD3_ACT_tIvtrDcRail1/1
  AWR 3 TX1/25 -> hvs_EMD3_ACT_tIvtrAcRailIphaSnsr1/1
  AWR 3 TX1/26 -> hvs_EMD3_ACT_tIvtrDcRailCnctr1/1
  AWR 3 TX1/27 -> hvs_EMD3_ACT_tCoolIvtrOuttk1/1
  Bus Selector22/1 -> AWR 1 TX1/1  "<EMD1_ACT_DcLinkVoltage>"
  Bus Selector22/2 -> AWR 1 TX1/2  "<EMD_ACT_DigitalInput1>"
  Bus Selector22/3 -> AWR 1 TX1/3  "<EMD_ACT_MaximumAvailableTorque>"
  Bus Selector22/4 -> AWR 1 TX1/4  "<EMD_ACT_DcLinkPower>"
  Bus Selector22/5 -> AWR 1 TX1/5  "<EMD_ACT_MotorSpeed>"
  Bus Selector22/6 -> AWR 1 TX1/6  "<EMD_ACT_MotorTorque>"
  Bus Selector22/7 -> AWR 1 TX1/7  "<EMD_ACT_InverterState>"
  Bus Selector22/8 -> AWR 1 TX1/8  "<EMD_ACT_ReferenceTorqueLimited>"
  Bus Selector22/9 -> AWR 1 TX1/9  "<drvEmot_T_Stator>"
  Bus Selector22/10 -> AWR 1 TX1/10  "<drvEmot_T_Rotor>"
  Bus Selector22/11 -> AWR 1 TX1/11  "<Inv_Ploss>"
  Bus Selector22/12 -> AWR 1 TX1/12  "<mot_Ploss>"
  Bus Selector22/13 -> AWR 1 TX1/13  "<uStator>"
  Bus Selector22/14 -> AWR 1 TX1/14  "<iStator>"
  Bus Selector26/1 -> AWR 1 TX1/17  "driveInverter_Temperatures_Bus"
  AWR 1 TX1/1 -> hvs_EMD1_ACT_DigitalInput2/1
  AWR 1 TX1/2 -> hvs_EMD1_ACT_InverterState1/1
  AWR 1 TX1/3 -> hvs_EMD1_ACT_MaxAvailableTorque1/1
  AWR 1 TX1/4 -> hvs_EMD1_ACT_ReferenceTorqueLim1/1
  AWR 1 TX1/5 -> hvs_EMD1_ACT_Torque1/1
  AWR 1 TX1/6 -> hvs_EMD1_ACT_DcLinkPower1/1
  AWR 1 TX1/7 -> hvs_EMD1_ACT_MotorSpeed1/1
  AWR 1 TX1/8 -> hvs_EMD1_ACT_DcLinkVoltage1/1
  AWR 1 TX1/9 -> hvs_EMD1_ACT_MotorTemperature1/1
  AWR 1 TX1/10 -> hvs_EMD1_ACT_RotorTemperature1/1
  AWR 1 TX1/11 -> hvs_EMD1_ACT_InverterLosses1/1
  AWR 1 TX1/12 -> hvs_EMD1_ACT_MotorLosses1/1
  AWR 1 TX1/13 -> hvs_EMD1_uStator1/1
  AWR 1 TX1/14 -> hvs_EMD1_iStator1/1
  AWR 1 TX1/17 -> hvs_EMD1_ACT_MaxJunctionTemp1/1
  AWR 1 TX1/18 -> hvs_EMD1_ACT_tSnsrPwrModlMax1/1
  AWR 1 TX1/19 -> hvs_EMD1_ACT_tCapSnsr1/1
  AWR 1 TX1/20 -> hvs_EMD1_ACT_tCapCoil1/1
  AWR 1 TX1/21 -> hvs_EMD1_ACT_tCapAcCnctr1/1
  AWR 1 TX1/22 -> hvs_EMD1_ACT_tCapDcCnctr1/1
  AWR 1 TX1/23 -> hvs_EMD1_ACT_tIvtrAcRail1/1
  AWR 1 TX1/24 -> hvs_EMD1_ACT_tIvtrDcRail1/1
  AWR 1 TX1/25 -> hvs_EMD1_ACT_tIvtrAcRailIphaSnsr1/1
  AWR 1 TX1/26 -> hvs_EMD1_ACT_tIvtrDcRailCnctr1/1
  AWR 1 TX1/27 -> hvs_EMD1_ACT_tCoolIvtrOuttk1/1
  Bus Selector23/1 -> AWR 4 TX1/1  "<EMD4_ACT_DcLinkVoltage>"
  Bus Selector23/2 -> AWR 4 TX1/2  "<EMD_ACT_DigitalInput1>"
  Bus Selector23/3 -> AWR 4 TX1/3  "<EMD_ACT_MaximumAvailableTorque>"
  Bus Selector23/4 -> AWR 4 TX1/4  "<EMD_ACT_DcLinkPower>"
  Bus Selector23/5 -> AWR 4 TX1/5  "<EMD_ACT_MotorSpeed>"
  Bus Selector23/6 -> AWR 4 TX1/6  "<EMD_ACT_MotorTorque>"
  Bus Selector23/7 -> AWR 4 TX1/7  "<EMD_ACT_InverterState>"
  Bus Selector23/8 -> AWR 4 TX1/8  "<EMD_ACT_ReferenceTorqueLimited>"
  Bus Selector23/9 -> AWR 4 TX1/9  "<drvEmot_T_Stator>"
  Bus Selector23/10 -> AWR 4 TX1/10  "<drvEmot_T_Rotor>"
  Bus Selector23/11 -> AWR 4 TX1/11  "<Inv_Ploss>"
  Bus Selector23/12 -> AWR 4 TX1/12  "<mot_Ploss>"
  Bus Selector23/13 -> AWR 4 TX1/13  "<uStator>"
  Bus Selector23/14 -> AWR 4 TX1/14  "<iStator>"
  Bus Selector27/1 -> AWR 4 TX1/17  "driveInverter_Temperatures_Bus"
  AWR 4 TX1/1 -> hvs_EMD4_ACT_DigitalInput2/1
  AWR 4 TX1/2 -> hvs_EMD4_ACT_InverterState1/1
  AWR 4 TX1/3 -> hvs_EMD4_ACT_MaxAvailableTorque1/1
  AWR 4 TX1/4 -> hvs_EMD4_ACT_ReferenceTorqueLim1/1
  AWR 4 TX1/5 -> hvs_EMD4_ACT_Torque1/1
  AWR 4 TX1/6 -> hvs_EMD4_ACT_DcLinkPower1/1
  AWR 4 TX1/7 -> hvs_EMD4_ACT_MotorSpeed1/1
  AWR 4 TX1/8 -> hvs_EMD4_ACT_DcLinkVoltage1/1
  AWR 4 TX1/9 -> hvs_EMD4_ACT_MotorTemperature1/1
  AWR 4 TX1/10 -> hvs_EMD4_ACT_RotorTemperature1/1
  AWR 4 TX1/11 -> hvs_EMD4_ACT_InverterLosses1/1
  AWR 4 TX1/12 -> hvs_EMD4_ACT_MotorLosses1/1
  AWR 4 TX1/13 -> hvs_EMD4_uStator1/1
  AWR 4 TX1/14 -> hvs_EMD4_iStator1/1
  AWR 4 TX1/17 -> hvs_EMD4_ACT_MaxJunctionTemperature1/1
  AWR 4 TX1/18 -> hvs_EMD4_ACT_tSnsrPwrModlMax1/1
  AWR 4 TX1/19 -> hvs_EMD4_ACT_tCapSnsr1/1
  AWR 4 TX1/20 -> hvs_EMD4_ACT_tCapCoil1/1
  AWR 4 TX1/21 -> hvs_EMD4_ACT_tCapAcCnctr1/1
  AWR 4 TX1/22 -> hvs_EMD4_ACT_tCapDcCnctr1/1
  AWR 4 TX1/23 -> hvs_EMD4_ACT_tIvtrAcRail1/1
  AWR 4 TX1/24 -> hvs_EMD4_ACT_tIvtrDcRail1/1
  AWR 4 TX1/25 -> hvs_EMD4_ACT_tIvtrAcRailIphaSnsr1/1
  AWR 4 TX1/26 -> hvs_EMD4_ACT_tIvtrDcRailCnctr1/1
  AWR 4 TX1/27 -> hvs_EMD4_ACT_tCoolIvtrOuttk1/1
  Bus Selector21/15 -> AWR 2 TX1/15  "<modIdx>"
  Bus Selector21/16 -> AWR 2 TX1/16  "<cosPhi>"
  AWR 2 TX1/15 -> hvs_EMD2_modIdx1/1
  AWR 2 TX1/16 -> hvs_EMD2_cosPhi1/1
  Bus Selector23/15 -> AWR 4 TX1/15  "<modIdx>"
  Bus Selector23/16 -> AWR 4 TX1/16  "<cosPhi>"
  AWR 4 TX1/16 -> hvs_EMD4_cosPhi1/1
  AWR 4 TX1/15 -> hvs_EMD4_modIdx1/1
  AWR 1 TX1/15 -> hvs_EMD1_modIdx1/1
  AWR 1 TX1/16 -> hvs_EMD1_cosPhi1/1
  Bus Selector22/15 -> AWR 1 TX1/15  "<modIdx>"
  Bus Selector22/16 -> AWR 1 TX1/16  "<cosPhi>"
  AWR 3 TX1/15 -> hvs_EMD3_modIdx1/1
  AWR 3 TX1/16 -> hvs_EMD3_cosPhi1/1
  Bus Selector28/15 -> AWR 3 TX1/15  "<modIdx>"
  Bus Selector28/16 -> AWR 3 TX1/16  "<cosPhi>"
  AWR 2 TX1/28 -> hvs_EMD2_ACT_Torque_Nm1/1
  AWR 3 TX1/28 -> hvs_EMD3_ACT_Torque_Nm1/1
  AWR 1 TX1/28 -> hvs_EMD1_ACT_Torque_Nm1/1
  AWR 4 TX1/28 -> hvs_EMD4_ACT_Torque_Nm1/1
  Bus Selector21/17 -> AWR 2 TX1/18  "<wasteHeat_coolant>"
  Bus Selector21/18 -> AWR 2 TX1/19  "<wasteHeat_oil>"
  Bus Selector28/17 -> AWR 3 TX1/18  "<wasteHeat_oil>"
  Bus Selector28/18 -> AWR 3 TX1/19  "<wasteHeat_coolant>"
  Bus Selector22/17 -> AWR 1 TX1/18  "<wasteHeat_coolant>"
  Bus Selector22/18 -> AWR 1 TX1/19  "<wasteHeat_oil>"
  Bus Selector23/17 -> AWR 4 TX1/18  "<wasteHeat_coolant>"
  Bus Selector23/18 -> AWR 4 TX1/19  "<wasteHeat_oil>"
  AWR 2 TX1/30 -> hvs_drvEmot2WasteHeatoil_power/1
  AWR 2 TX1/29 -> hvs_drvEmot2WasteHeatcoolant_power/1
  AWR 3 TX1/30 -> hvs_drvEmot3WasteHeatoil_power/1
  AWR 3 TX1/29 -> hvs_drvEmot3WasteHeatcoolant_power/1
  AWR 1 TX1/29 -> hvs_drvEmot1WasteHeatcoolant_power/1
  AWR 1 TX1/30 -> hvs_drvEmot1WasteHeatoil_power/1
  AWR 4 TX1/29 -> hvs_drvEmot4WasteHeatcoolant_power/1
  AWR 4 TX1/30 -> hvs_drvEmot4WasteHeatoil_power/1

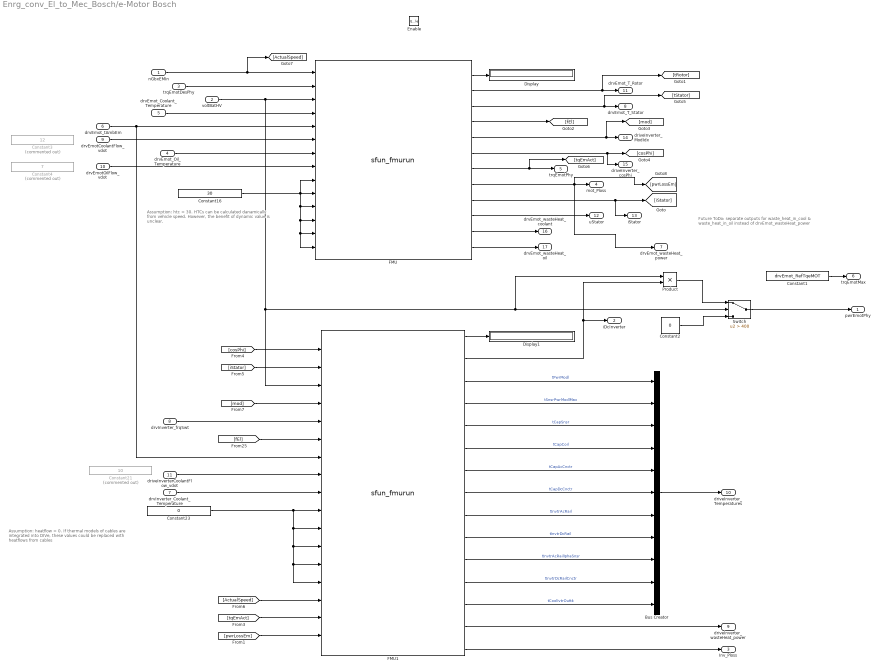
== system Enrg_conv_El_to_Mec_Bosch/e-Motor Bosch ==
  note: Assumption: heatflow = 0.
      | If thermal models of cables are integrated into DIVe, these values could be replaced with heatflows from cables
  note: Assumption: htc = 30.
      | HTCs can be calculated danamically from vehicle speed.
      | However, the benefit of dynamic value is unclear.
  note: Future ToDo:
      |
      | separate outputs for waste_heat_in_cool & waste_heat_in_oil instead of drvEmot_wasteHeat_power
  nGbxEMIn : Inport
  voltBatHV : Inport  Port=2
  trqEmotDesPhy : Inport  Port=3
  drvEmot_Oil_Temperature : Inport  Port=4
  drvEmot_Coolant_Temperature : Inport  Port=5
  drvEmot_tAmbEm : Inport  Port=6
  drvInverter_Coolant_Temperature : Inport  Port=7
  drvInverter_frqSwt : Inport  Port=8
  drvEmotCoolantFlow_vdot : Inport  Port=9
  drvEmotOilFlow_vdot : Inport  Port=10
  driveInverterCoolantFlow_vdot : Inport  Port=11
  Enable : EnablePort
  Bus Creator : BusCreator  Inputs=11
  Constant1 : Constant  Value=drvEmot_RefTqeMOT
  Constant16 : Constant  Value=30
  Constant2 : Constant  Value=0
  Constant21 : Constant  Commented=on  Value=10
  Constant23 : Constant  Value=0
  Constant3 : Constant  Commented=on  Value=12
  Constant4 : Constant  Commented=on  Value=7
  Display : Display
      settings: Format=binary (Stored Integer)
  Display1 : Display
      settings: Format=binary (Stored Integer)
  FMU : S-Function  LoadFcn=FMIKit.setSFunctionParameters(gcb)  FunctionName=sfun_fmurun  Parameters='2.0' 1 '{2113429a-3421-43ca-bf64-113b3d614243}' 'PSM431_582_DAI_Truck' FMIKit.getUnzipDirectory(gcb) 0 0 0 '' 0 -1 0 0 0 [] [] [] [] char({}) [1 1 1 1 1 1 1 1 1 1 1 1 1 1] [0 0 0 0 0 0 0 0 0 0 0 0 0 0] [0 0 0 0 0 0 0 0 0 0 0 0 0 0] [2 3 4 5 6 7 8 9 10 11 12 13 14 15] [1 1 1 1 1 1 1 1 1 1 1 1] [1 0 0 0 0 0 0 0 0 0 0 0] [16 17 18 19 20 21 22 23 24 25 26 27]  SFunctionDeploymentMode=off  EnableBusSupport=off
      settings: DeleteFcn=FMIKit.closeBlockDialog(gcbh)  ModelCloseFcn=FMIKit.closeBlockDialog(gcbh)  DestroyFcn=FMIKit.closeBlockDialog(gcbh)  OpenFcn=FMIKit.showBlockDialog(gcbh);  CloseFcn=FMIKit.closeBlockDialog(gcbh)  ParentCloseFcn=FMIKit.closeBlockDialog(gcbh)
      mask Help: eval('FMIKit.showBlockDialogHelp();')
      mask Display:
      | ports = get_param(gcb, 'Ports');
      | 
      | inports = FMIKit.getInportLabels(gcb);
      | 
      | for i = 1:min(numel(inports), ports(1))
      |     port_label('input', i, inports{i})
      | end
      | 
      | outports = FMIKit.getOutportLabels(gcb);
      | 
      | for i = 1:min(numel(outports), ports(2))
      |     port_label('output', i, outports{i})
      | end
      | 
      | if isempty(inports) && isempty(outports)
      |     patch([-20 65, 65 -20], [-20 -20 70 70], [1 1 1])
      |     plot([-2 50 50 -2 -2], [0 0 50 50 0])
      |     patch([-9 12 12 -9 -9], [12 12 20 20 12], [1 1 1])
      |     plot([-9 12 12 -9 -9], [12 12 20 20 12])
      |     patch([-9 12 12 -9 -9], [30 30 38 38 30], [1 1 1])
      |     plot([-9 12 12 -9 -9], [30 30 38 38 30])
      | end
  FMU1 : S-Function  LoadFcn=FMIKit.setSFunctionParameters(gcb)  FunctionName=sfun_fmurun  Parameters='2.0' 1 '{21300c3e-3412-4298-b3f8-faa2125208c1}' 'Ivtr_Gen4FL_600A_DAI_C0_V3' FMIKit.getUnzipDirectory(gcb) 0 0 0 '' 0 -1 0 0 0 [] [] [] [] char({}) [1 1 1 1 1 1 1 1 1 1 1 1 1 1 1 1 1] [0 0 0 0 0 0 0 0 0 0 0 0 0 0 0 0 0] [0 0 0 0 0 0 0 0 0 0 0 0 0 0 0 0 0] [3 4 5 6 7 8 9 10 11 12 13 14 15 16 17 18 19] [1 1 1 1 1 1 1 1 1 1 1 1 1 1 1] [1 0 0 0 0 0 0 0 0 0 0 0 0 0 0] [20 21 22 23 24 25 26 27 28 29 30 31 32 33 34]  SFunctionDeploymentMode=off  EnableBusSupport=off
      settings: DeleteFcn=FMIKit.closeBlockDialog(gcbh)  ModelCloseFcn=FMIKit.closeBlockDialog(gcbh)  DestroyFcn=FMIKit.closeBlockDialog(gcbh)  OpenFcn=FMIKit.showBlockDialog(gcbh);  CloseFcn=FMIKit.closeBlockDialog(gcbh)  ParentCloseFcn=FMIKit.closeBlockDialog(gcbh)
      mask Help: eval('FMIKit.showBlockDialogHelp();')
      mask Display:
      | ports = get_param(gcb, 'Ports');
      | 
      | inports = FMIKit.getInportLabels(gcb);
      | 
      | for i = 1:min(numel(inports), ports(1))
      |     port_label('input', i, inports{i})
      | end
      | 
      | outports = FMIKit.getOutportLabels(gcb);
      | 
      | for i = 1:min(numel(outports), ports(2))
      |     port_label('output', i, outports{i})
      | end
      | 
      | if isempty(inports) && isempty(outports)
      |     patch([-20 65, 65 -20], [-20 -20 70 70], [1 1 1])
      |     plot([-2 50 50 -2 -2], [0 0 50 50 0])
      |     patch([-9 12 12 -9 -9], [12 12 20 20 12], [1 1 1])
      |     plot([-9 12 12 -9 -9], [12 12 20 20 12])
      |     patch([-9 12 12 -9 -9], [30 30 38 38 30], [1 1 1])
      |     plot([-9 12 12 -9 -9], [30 30 38 38 30])
      | end
  Product : Product
  Switch : Switch  Criteria=u2 > Threshold  Threshold=400
  pwrEmotPhy : Outport
  iDcInverter : Outport  Port=2
  Inv_Ploss : Outport  Port=3
  mot_Ploss : Outport  Port=4
  trqEmotPhy : Outport  Port=5
  trqEmotMax : Outport  Port=6
  drvEmot_wasteHeat_power : Outport  Port=7
  drvEmot_T_Stator : Outport  Port=8
  driveInverter_wasteHeat_power : Outport  Port=9
  driveInverter_Temperatures : Outport  Port=10
  drvEmot_T_Rotor : Outport  Port=11
  uStator : Outport  Port=12
  iStator : Outport  Port=13
  driveInverter_ModIdx : Outport  Port=14
  driveInverter_cosPhi : Outport  Port=15
  drvEmot_wasteHeat_coolant : Outport  Port=16
  drvEmot_wasteHeat_oil : Outport  Port=17
  wires:
  FMU/4 -> [fEl]
  FMU/8 -> drvEmot_wasteHeat_power/1, [pwrLossEm], mot_Ploss/1
  FMU1/4 -> Bus Creator/2  "tSnsrPwrModlMax"
  FMU1/10 -> Bus Creator/8  "tInvtrDcRail"
  drvEmotCoolantFlow_vdot/1 -> FMU/6
  [mod] -> FMU1/4
  FMU1/5 -> Bus Creator/3  "tCapSnsr"
  [cosPhi] -> FMU1/1
  FMU/5 -> driveInverter_ModIdx/1, [mod]
  drvEmot_tAmbEm/1 -> FMU1/7, FMU/5
  [iStator] -> FMU1/2
  drvEmotOilFlow_vdot/1 -> FMU/8
  FMU1/12 -> Bus Creator/10  "tInvtrDcRailCnctr"
  FMU1/8 -> Bus Creator/6  "tCapDcCnctr"
  FMU/6 -> driveInverter_cosPhi/1, [cosPhi]
  [fEl] -> FMU1/6
  FMU1/11 -> Bus Creator/9  "tInvtrAcRailIphaSnsr"
  FMU/2 -> [tRotor], drvEmot_T_Rotor/1
  FMU1/6 -> Bus Creator/4  "tCapCoil"
  drvInverter_frqSwt/1 -> FMU1/5
  Bus Creator/1 -> driveInverter_Temperatures/1
  FMU1/7 -> Bus Creator/5  "tCapAcCnctr"
  FMU1/13 -> Bus Creator/11  "tCoolIvtrOuttk"
  FMU/3 -> [tStator], drvEmot_T_Stator/1
  FMU/7 -> [tqEmAct], trqEmotPhy/1
  FMU1/9 -> Bus Creator/7  "tInvtrAcRail"
  trqEmotDesPhy/1 -> FMU/2
  FMU/10 -> uStator/1
  FMU/9 -> [iStator], iStator/1
  Constant1/1 -> trqEmotMax/1
  Product/1 -> Switch/1
  Switch/1 -> pwrEmotPhy/1
  Constant2/1 -> Switch/3
  voltBatHV/1 -> FMU/3, FMU1/3, Product/1, Switch/2
  FMU1/3 -> Bus Creator/1  "tPwrModl"
  FMU1/2 -> Product/2, iDcInverter/1
  nGbxEMIn/1 -> FMU/1, [ActualSpeed]
  drvEmot_Coolant_Temperature/1 -> FMU/4
  drvEmot_Oil_Temperature/1 -> FMU/7
  drvInverter_Coolant_Temperature/1 -> FMU1/9
  FMU1/15 -> Inv_Ploss/1
  FMU1/14 -> driveInverter_wasteHeat_power/1
  driveInverterCoolantFlow_vdot/1 -> FMU1/8
  FMU/1 -> Display/1
  FMU1/1 -> Display1/1
  [tqEmAct] -> FMU1/16
  [ActualSpeed] -> FMU1/15
  FMU/12 -> drvEmot_wasteHeat_oil/1
  FMU/11 -> drvEmot_wasteHeat_coolant/1
  Constant16/1 -> FMU/12, FMU/13, FMU/14, FMU/11, FMU/9, FMU/10
  [pwrLossEm] -> FMU1/17
  Constant23/1 -> FMU1/11, FMU1/12, FMU1/13, FMU1/14, FMU1/10

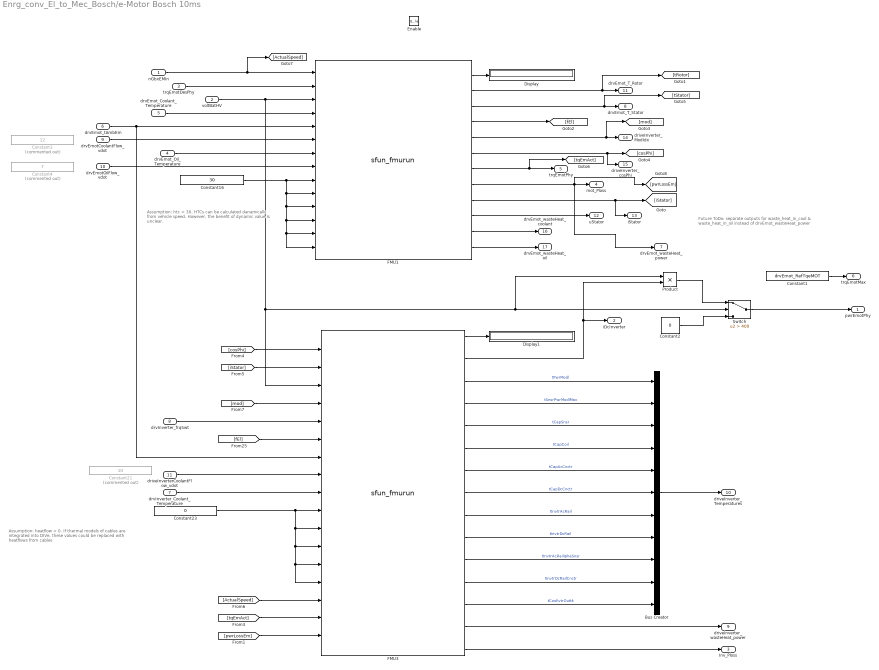
== system Enrg_conv_El_to_Mec_Bosch/e-Motor Bosch 10ms ==
  note: Assumption: heatflow = 0.
      | If thermal models of cables are integrated into DIVe, these values could be replaced with heatflows from cables
  note: Assumption: htc = 30.
      | HTCs can be calculated danamically from vehicle speed.
      | However, the benefit of dynamic value is unclear.
  note: Future ToDo:
      |
      | separate outputs for waste_heat_in_cool & waste_heat_in_oil instead of drvEmot_wasteHeat_power
  nGbxEMIn : Inport
  voltBatHV : Inport  Port=2
  trqEmotDesPhy : Inport  Port=3
  drvEmot_Oil_Temperature : Inport  Port=4
  drvEmot_Coolant_Temperature : Inport  Port=5
  drvEmot_tAmbEm : Inport  Port=6
  drvInverter_Coolant_Temperature : Inport  Port=7
  drvInverter_frqSwt : Inport  Port=8
  drvEmotCoolantFlow_vdot : Inport  Port=9
  drvEmotOilFlow_vdot : Inport  Port=10
  driveInverterCoolantFlow_vdot : Inport  Port=11
  Enable : EnablePort
  Bus Creator : BusCreator  Inputs=11
  Constant1 : Constant  Value=drvEmot_RefTqeMOT
  Constant16 : Constant  Value=30
  Constant2 : Constant  Value=0
  Constant21 : Constant  Commented=on  Value=10
  Constant23 : Constant  Value=0
  Constant3 : Constant  Commented=on  Value=12
  Constant4 : Constant  Commented=on  Value=7
  Display : Display
      settings: Format=binary (Stored Integer)
  Display1 : Display
      settings: Format=binary (Stored Integer)
  FMU1 : S-Function  LoadFcn=FMIKit.setSFunctionParameters(gcb)  FunctionName=sfun_fmurun  Parameters='2.0' 1 '{a1d13a0a-31d4-402f-bb1d-574e579b5687}' 'PSM431_582_DAI_Truck' FMIKit.getUnzipDirectory(gcb) 0 0 0 '' 0 -1 0 0 0 [] [] [] [] char({}) [1 1 1 1 1 1 1 1 1 1 1 1 1 1] [0 0 0 0 0 0 0 0 0 0 0 0 0 0] [0 0 0 0 0 0 0 0 0 0 0 0 0 0] [2 3 4 5 6 7 8 9 10 11 12 13 14 15] [1 1 1 1 1 1 1 1 1 1 1 1] [1 0 0 0 0 0 0 0 0 0 0 0] [16 17 18 19 20 21 22 23 24 25 26 27]  SFunctionDeploymentMode=off  EnableBusSupport=off
      settings: DeleteFcn=FMIKit.closeBlockDialog(gcbh)  ModelCloseFcn=FMIKit.closeBlockDialog(gcbh)  DestroyFcn=FMIKit.closeBlockDialog(gcbh)  OpenFcn=FMIKit.showBlockDialog(gcbh);  CloseFcn=FMIKit.closeBlockDialog(gcbh)  ParentCloseFcn=FMIKit.closeBlockDialog(gcbh)
      mask Help: eval('FMIKit.showBlockDialogHelp();')
      mask Display:
      | ports = get_param(gcb, 'Ports');
      | 
      | inports = FMIKit.getInportLabels(gcb);
      | 
      | for i = 1:min(numel(inports), ports(1))
      |     port_label('input', i, inports{i})
      | end
      | 
      | outports = FMIKit.getOutportLabels(gcb);
      | 
      | for i = 1:min(numel(outports), ports(2))
      |     port_label('output', i, outports{i})
      | end
      | 
      | if isempty(inports) && isempty(outports)
      |     patch([-20 65, 65 -20], [-20 -20 70 70], [1 1 1])
      |     plot([-2 50 50 -2 -2], [0 0 50 50 0])
      |     patch([-9 12 12 -9 -9], [12 12 20 20 12], [1 1 1])
      |     plot([-9 12 12 -9 -9], [12 12 20 20 12])
      |     patch([-9 12 12 -9 -9], [30 30 38 38 30], [1 1 1])
      |     plot([-9 12 12 -9 -9], [30 30 38 38 30])
      | end
  FMU3 : S-Function  LoadFcn=FMIKit.setSFunctionParameters(gcb)  FunctionName=sfun_fmurun  Parameters='2.0' 1 '{23397740-028f-479d-abac-30f377e6905b}' 'Ivtr_Gen4FL_600A_DAI_C0_V3' FMIKit.getUnzipDirectory(gcb) 0 0 0 '' 0 -1 0 0 0 [] [] [] [] char({}) [1 1 1 1 1 1 1 1 1 1 1 1 1 1 1 1 1] [0 0 0 0 0 0 0 0 0 0 0 0 0 0 0 0 0] [0 0 0 0 0 0 0 0 0 0 0 0 0 0 0 0 0] [3 4 5 6 7 8 9 10 11 12 13 14 15 16 17 18 19] [1 1 1 1 1 1 1 1 1 1 1 1 1 1 1] [1 0 0 0 0 0 0 0 0 0 0 0 0 0 0] [20 21 22 23 24 25 26 27 28 29 30 31 32 33 34]  SFunctionDeploymentMode=off  EnableBusSupport=off
      settings: DeleteFcn=FMIKit.closeBlockDialog(gcbh)  ModelCloseFcn=FMIKit.closeBlockDialog(gcbh)  DestroyFcn=FMIKit.closeBlockDialog(gcbh)  OpenFcn=FMIKit.showBlockDialog(gcbh);  CloseFcn=FMIKit.closeBlockDialog(gcbh)  ParentCloseFcn=FMIKit.closeBlockDialog(gcbh)
      mask Help: eval('FMIKit.showBlockDialogHelp();')
      mask Display:
      | ports = get_param(gcb, 'Ports');
      | 
      | inports = FMIKit.getInportLabels(gcb);
      | 
      | for i = 1:min(numel(inports), ports(1))
      |     port_label('input', i, inports{i})
      | end
      | 
      | outports = FMIKit.getOutportLabels(gcb);
      | 
      | for i = 1:min(numel(outports), ports(2))
      |     port_label('output', i, outports{i})
      | end
      | 
      | if isempty(inports) && isempty(outports)
      |     patch([-20 65, 65 -20], [-20 -20 70 70], [1 1 1])
      |     plot([-2 50 50 -2 -2], [0 0 50 50 0])
      |     patch([-9 12 12 -9 -9], [12 12 20 20 12], [1 1 1])
      |     plot([-9 12 12 -9 -9], [12 12 20 20 12])
      |     patch([-9 12 12 -9 -9], [30 30 38 38 30], [1 1 1])
      |     plot([-9 12 12 -9 -9], [30 30 38 38 30])
      | end
  Product : Product
  Switch : Switch  Criteria=u2 > Threshold  Threshold=400
  pwrEmotPhy : Outport
  iDcInverter : Outport  Port=2
  Inv_Ploss : Outport  Port=3
  mot_Ploss : Outport  Port=4
  trqEmotPhy : Outport  Port=5
  trqEmotMax : Outport  Port=6
  drvEmot_wasteHeat_power : Outport  Port=7
  drvEmot_T_Stator : Outport  Port=8
  driveInverter_wasteHeat_power : Outport  Port=9
  driveInverter_Temperatures : Outport  Port=10
  drvEmot_T_Rotor : Outport  Port=11
  uStator : Outport  Port=12
  iStator : Outport  Port=13
  driveInverter_ModIdx : Outport  Port=14
  driveInverter_cosPhi : Outport  Port=15
  drvEmot_wasteHeat_coolant : Outport  Port=16
  drvEmot_wasteHeat_oil : Outport  Port=17
  wires:
  FMU1/4 -> [fEl]
  FMU1/8 -> drvEmot_wasteHeat_power/1, [pwrLossEm], mot_Ploss/1
  FMU3/4 -> Bus Creator/2  "tSnsrPwrModlMax"
  FMU3/10 -> Bus Creator/8  "tInvtrDcRail"
  drvEmotCoolantFlow_vdot/1 -> FMU1/6
  [mod] -> FMU3/4
  FMU3/5 -> Bus Creator/3  "tCapSnsr"
  [cosPhi] -> FMU3/1
  FMU1/5 -> driveInverter_ModIdx/1, [mod]
  drvEmot_tAmbEm/1 -> FMU3/7, FMU1/5
  [iStator] -> FMU3/2
  drvEmotOilFlow_vdot/1 -> FMU1/8
  FMU3/12 -> Bus Creator/10  "tInvtrDcRailCnctr"
  FMU3/8 -> Bus Creator/6  "tCapDcCnctr"
  FMU1/6 -> driveInverter_cosPhi/1, [cosPhi]
  [fEl] -> FMU3/6
  FMU3/11 -> Bus Creator/9  "tInvtrAcRailIphaSnsr"
  FMU1/2 -> [tRotor], drvEmot_T_Rotor/1
  FMU3/6 -> Bus Creator/4  "tCapCoil"
  drvInverter_frqSwt/1 -> FMU3/5
  Bus Creator/1 -> driveInverter_Temperatures/1
  FMU3/7 -> Bus Creator/5  "tCapAcCnctr"
  FMU3/13 -> Bus Creator/11  "tCoolIvtrOuttk"
  FMU1/3 -> [tStator], drvEmot_T_Stator/1
  FMU1/7 -> [tqEmAct], trqEmotPhy/1
  FMU3/9 -> Bus Creator/7  "tInvtrAcRail"
  trqEmotDesPhy/1 -> FMU1/2
  FMU1/10 -> uStator/1
  FMU1/9 -> [iStator], iStator/1
  Constant1/1 -> trqEmotMax/1
  Product/1 -> Switch/1
  Switch/1 -> pwrEmotPhy/1
  Constant2/1 -> Switch/3
  voltBatHV/1 -> FMU1/3, FMU3/3, Product/1, Switch/2
  FMU3/3 -> Bus Creator/1  "tPwrModl"
  FMU3/2 -> Product/2, iDcInverter/1
  nGbxEMIn/1 -> FMU1/1, [ActualSpeed]
  drvEmot_Coolant_Temperature/1 -> FMU1/4
  drvEmot_Oil_Temperature/1 -> FMU1/7
  drvInverter_Coolant_Temperature/1 -> FMU3/9
  FMU3/15 -> Inv_Ploss/1
  FMU3/14 -> driveInverter_wasteHeat_power/1
  driveInverterCoolantFlow_vdot/1 -> FMU3/8
  FMU1/1 -> Display/1
  FMU3/1 -> Display1/1
  [tqEmAct] -> FMU3/16
  [ActualSpeed] -> FMU3/15
  FMU1/12 -> drvEmot_wasteHeat_oil/1
  FMU1/11 -> drvEmot_wasteHeat_coolant/1
  Constant16/1 -> FMU1/10, FMU1/11, FMU1/12, FMU1/13, FMU1/14, FMU1/9
  Constant23/1 -> FMU3/13, FMU3/14, FMU3/12, FMU3/11, FMU3/10
  [pwrLossEm] -> FMU3/17
